simulink model "HPOP"  (R2023a)
settings: Solver=ode4  StartTime=0.0  StopTime=10.0  FixedStep=6000  RelTol=1e-3
undefined symbols (not defined in the file or in its folder): plant
settings Model: Creator=ndelurgio  LastModifiedBy=ndelurgio

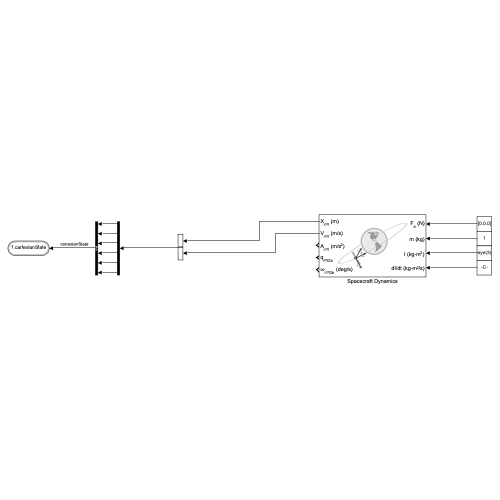
[thumbnail: Simulink's stored preview of the top-level diagram]
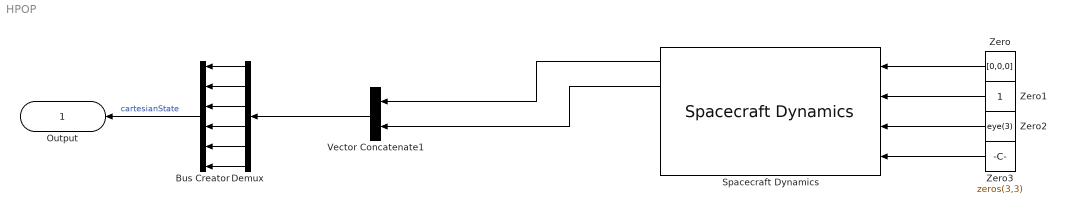
== system HPOP ==
  Bus Creator : BusCreator  Inputs=6  OutDataTypeStr=Bus: cartesianState  NonVirtualBus=on
      settings: InheritFromInputs=off
  Demux : Demux  Outputs=6
  Spacecraft Dynamics : SpacecraftDynamics  momentsIn=off  outputAccel=on  dateOut=off  massType=Custom variable  stateFormatNum=ICRF state vector  inertialPosition=[plant.chief.initialConditions.cartesianState.positionX_J2000_m,plant.chief.initialConditions.cartesianState.positionY_J2000_m,plant.chief.initialConditions.cartesianState.positionZ_J2000_m]  inertialVelocity=[plant.chief.initialConditions.cartesianState.velocityX_J2000_m,plant.chief.initialConditions.cartesianState.velocityY_J2000_m,plant.chief.initialConditions.cartesianState.velocityZ_J2000_m]  useGravGrad=off  gravityModel=Oblate ellipsoid (J2)  useEOPs=off
  Vector Concatenate1 : Concatenate
  Zero : Constant  Value=[0,0,0]  OutDataTypeStr=Inherit: Inherit via back propagation
  Zero1 : Constant  OutDataTypeStr=Inherit: Inherit via back propagation
  Zero2 : Constant  Value=eye(3)  OutDataTypeStr=Inherit: Inherit via back propagation
  Zero3 : Constant  Value=zeros(3,3)  OutDataTypeStr=Inherit: Inherit via back propagation
  Output : Outport  OutDataTypeStr=Bus: cartesianState  BusOutputAsStruct=on
  wires:
  Zero/1 -> Spacecraft Dynamics/1
  Zero1/1 -> Spacecraft Dynamics/2
  Zero2/1 -> Spacecraft Dynamics/3
  Zero3/1 -> Spacecraft Dynamics/4
  Spacecraft Dynamics/2 -> Vector Concatenate1/2
  Spacecraft Dynamics/1 -> Vector Concatenate1/1
  Demux/3 -> Bus Creator/3
  Bus Creator/1 -> Output/1  "cartesianState"
  Demux/6 -> Bus Creator/6
  Demux/1 -> Bus Creator/1
  Demux/4 -> Bus Creator/4
  Demux/2 -> Bus Creator/2
  Demux/5 -> Bus Creator/5
  Vector Concatenate1/1 -> Demux/1
